simulink model "pendulum"  (R2019a)
settings: Solver=VariableStepAuto  StartTime=0.0  StopTime=tfinal  MaxStep=tstepmax  RelTol=1e-3
values from neighbouring files (symbols this model uses):
  c = 0.5    [pendulumscript.m]
  g = 10    [pendulumscript.m]
  L = 1    [pendulumscript.m]
  m = 1    [pendulumscript.m]
  thetha0 = 0* pi/180    (= 0)    [pendulumscript.m]
  thethadot0 = 0    [pendulumscript.m]
settings Model: Creator=Meet  LastModifiedBy=Meet

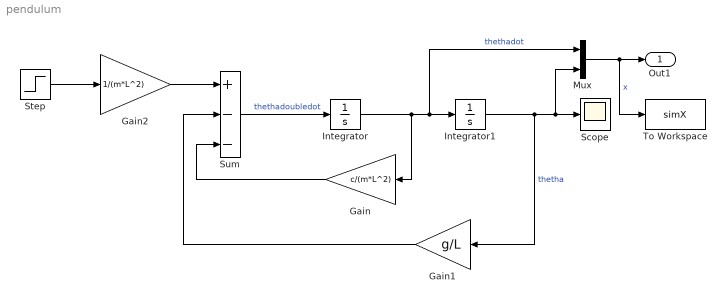
== system pendulum ==
  Gain : Gain  Gain=c/(m*L^2)
  Gain1 : Gain  Gain=g/L
  Gain2 : Gain  Gain=1/(m*L^2)
  Integrator : Integrator  InitialCondition=thethadot0
  Integrator1 : Integrator  InitialCondition=thetha0
  Mux : Mux  Inputs=2
  Scope : Scope
  Step : Step  Time=10  SampleTime=0
  Sum : Sum  Inputs=+--
  To Workspace : ToWorkspace  VariableName=simX  SaveFormat=Timeseries  SampleTime=-1
  Out1 : Outport
  wires:
  Step/1 -> Gain2/1
  Sum/1 -> Integrator/1  "thethadoubledot"
  Integrator/1 -> Mux/1, Integrator1/1, Gain/1  "thethadot"
  Integrator1/1 -> Mux/2, Scope/1, Gain1/1  "thetha"
  Gain/1 -> Sum/3
  Gain1/1 -> Sum/2
  Gain2/1 -> Sum/1
  Mux/1 -> To Workspace/1, Out1/1  "x"
